simulink model "metab_platform"  (Simulink 7.5)
settings: Solver=ode45  StartTime=0.0  StopTime=struttura.simul  FixedStep=0.5  MaxStep=1  RelTol=1e-3
undefined symbols (not defined in the file or in its folder): hardware, struttura
settings Model: Creator=Marc Breton  LastModifiedBy=sriddle
settings SolverCC: InitialStep=0.5
settings DataIOCC: ExternalInput=[t,u]  LimitDataPoints=off  SaveOutput=off  SignalLogging=off  SaveTime=off
settings OptimizationCC: InitFltsAndDblsToZero=on
settings DebuggingCC: SaveWithParameterizedLinksMsg=none  SignalResolutionControl=TryResolveAllWithWarning  InheritedTsInSrcMsg=none  MultiTaskDSMMsg=warning  MultiTaskCondExecSysMsg=none  StrictBusMsg=Warning
settings RTWCC: IncludeERTFirstTime=on
settings GRTTargetCC: TargetFcnLib=ansi_tfl_tmw.mat

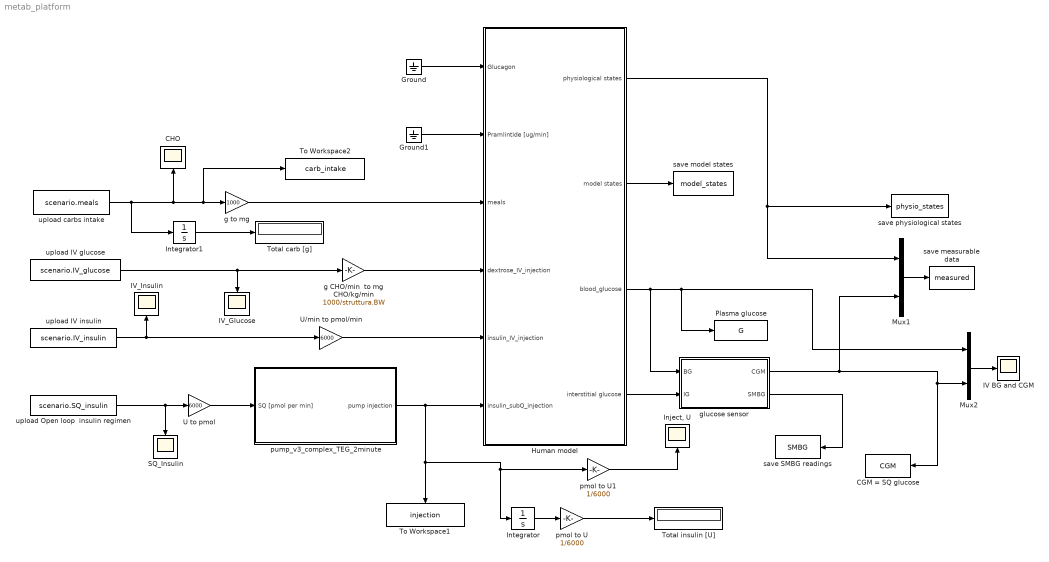
== system metab_platform ==
  CGM = SQ glucose : ToWorkspace  VariableName=CGM  SampleTime=-1  SaveFormat=Structure
  CHO : Scope
  Ground : Ground
  Ground1 : Ground
  Human model : Subsystem
  IV BG and CGM : Scope
      settings: YMin=0  YMax=3000
  IV_Glucose : Scope
      settings: YMin=-1  YMax=1  SaveName=ScopeData7
  IV_Insulin : Scope
      settings: YMin=-1  YMax=1  SaveName=ScopeData3
  "Inject, U" : Scope
      settings: SaveName=ScopeData2
  Integrator : Integrator
  Integrator1 : Integrator
  Mux1 : Mux  Inputs=2
  Mux2 : Mux  Inputs=2
  Plasma glucose : ToWorkspace  VariableName=G  SampleTime=-1  SaveFormat=Structure
  SQ_Insulin : Scope
      settings: SaveName=ScopeData6
  To Workspace1 : ToWorkspace  VariableName=injection  SampleTime=-1  SaveFormat=Structure
  To Workspace2 : ToWorkspace  VariableName=carb_intake  SampleTime=-1  SaveFormat=Structure
  Total carb [g] : Display
  Total insulin [U] : Display
  U to pmol : Gain  Gain=6000  ParameterDataType=sfix(16)  ParameterScaling=2^0  OutDataType=sfix(16)  OutScaling=2^0
  U/min to pmol/min : Gain  Gain=6000  ParameterDataType=sfix(16)  ParameterScaling=2^0  OutDataType=sfix(16)  OutScaling=2^0
  g CHO/min  to mg CHO/kg/min : Gain  Gain=1000/struttura.BW  ParameterDataType=sfix(16)  ParameterScaling=2^0  OutDataType=sfix(16)  OutScaling=2^0
  g to mg : Gain  Gain=1000  ParameterDataType=sfix(16)  ParameterScaling=2^0  OutDataType=sfix(16)  OutScaling=2^0
  glucose sensor : Subsystem
  pmol to U : Gain  Gain=1/6000  ParameterDataType=sfix(16)  ParameterScaling=2^0  OutDataType=sfix(16)  OutScaling=2^0
  pmol to U1 : Gain  Gain=1/6000  ParameterDataType=sfix(16)  ParameterScaling=2^0  OutDataType=sfix(16)  OutScaling=2^0
  pump_v3_complex_TEG_2minute : Subsystem
  save SMBG readings : ToWorkspace  VariableName=SMBG  SampleTime=-1  SaveFormat=Structure
  save measurable data : ToWorkspace  VariableName=measured  SampleTime=-1  SaveFormat=Structure
  save model states : ToWorkspace  VariableName=model_states  SampleTime=-1  SaveFormat=Structure With Time
  save physiological states : ToWorkspace  VariableName=physio_states  SampleTime=-1  SaveFormat=Structure With Time
  upload IV glucose : FromWorkspace  VariableName=scenario.IV_glucose  SampleTime=0
  upload IV insulin : FromWorkspace  VariableName=scenario.IV_insulin  SampleTime=0
  upload Open loop  insulin regimen : FromWorkspace  VariableName=scenario.SQ_insulin  SampleTime=0
  upload carbs intake : FromWorkspace  VariableName=scenario.meals  SampleTime=0
  wires:
  upload carbs intake/1 -> Integrator1/1, CHO/1, g to mg/1, To Workspace2/1
  g to mg/1 -> Human model/3(meals)
  upload Open loop  insulin regimen/1 -> U to pmol/1, SQ_Insulin/1
  U to pmol/1 -> pump_v3_complex_TEG_2minute/1(SQ [pmol per min])
  pump_v3_complex_TEG_2minute/1(pump injection) -> To Workspace1/1, Integrator/1, pmol to U1/1, Human model/6(insulin_subQ_injection)
  Integrator/1 -> pmol to U/1
  pmol to U/1 -> Total insulin [U]/1
  Integrator1/1 -> Total carb [g]/1
  upload IV glucose/1 -> g CHO/min  to mg CHO/kg/min/1, IV_Glucose/1
  upload IV insulin/1 -> U/min to pmol/min/1, IV_Insulin/1
  U/min to pmol/min/1 -> Human model/5(insulin_IV_injection)
  g CHO/min  to mg CHO/kg/min/1 -> Human model/4(dextrose_IV_injection)
  Human model/3(blood_glucose) -> Mux2/1, Plasma glucose/1, glucose sensor/1(BG)
  Human model/1(physiological states) -> Mux1/1, save physiological states/1
  Human model/2(model states) -> save model states/1
  Human model/4(interstitial glucose) -> glucose sensor/2(IG)
  Mux1/1 -> save measurable data/1
  glucose sensor/2(SMBG) -> save SMBG readings/1
  glucose sensor/1(CGM) -> Mux1/2, CGM = SQ glucose/1, Mux2/2
  Mux2/1 -> IV BG and CGM/1
  pmol to U1/1 -> "Inject, U"/1
  Ground/1 -> Human model/1(Glucagon)
  Ground1/1 -> Human model/2(Pramlintide [ug/min])

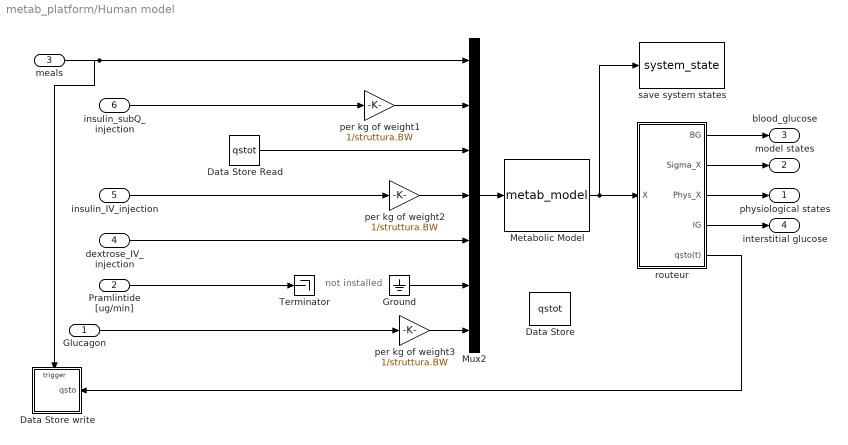
== system metab_platform/Human model ==
  note: not
      | installed
  Glucagon : Inport
  Pramlintide [ug/min] : Inport  Port=2
  meals : Inport  Port=3
  dextrose_IV_injection : Inport  Port=4
  insulin_IV_injection : Inport  Port=5
  insulin_subQ_injection : Inport  Port=6
  Data Store : DataStoreMemory  DataStoreName=qstot
  Data Store Read : DataStoreRead  DataStoreName=qstot  SampleTime=-1
  Data Store write : Subsystem  TreatAsAtomicUnit=on
  Ground : Ground
  Metabolic Model : S-Function  FunctionName=metab_model  Parameters=struttura  EnableBusSupport=off
  Mux2 : Mux  Inputs=7
  Terminator : Terminator
  per kg of weight1 : Gain  Gain=1/struttura.BW
  per kg of weight2 : Gain  Gain=1/struttura.BW
  per kg of weight3 : Gain  Gain=1/struttura.BW
  routeur : Subsystem
  save system states : ToWorkspace  VariableName=system_state  SampleTime=-1  SaveFormat=Structure With Time
  physiological states : Outport
  model states : Outport  Port=2
  blood_glucose : Outport  Port=3
  interstitial glucose : Outport  Port=4
  wires:
  Metabolic Model/1 -> routeur/1(X), save system states/1
  routeur/3(Phys_X) -> physiological states/1
  routeur/1(BG) -> blood_glucose/1
  insulin_subQ_injection/1 -> per kg of weight1/1
  Mux2/1 -> Metabolic Model/1
  routeur/2(Sigma_X) -> model states/1
  Data Store Read/1 -> Mux2/3
  routeur/4(IG) -> interstitial glucose/1
  per kg of weight1/1 -> Mux2/2
  insulin_IV_injection/1 -> per kg of weight2/1
  dextrose_IV_injection/1 -> Mux2/5
  routeur/5(qsto(t)) -> Data Store write/1(qsto)
  per kg of weight2/1 -> Mux2/4
  meals/1 -> Data Store write/Trigger, Mux2/1
  Pramlintide [ug/min]/1 -> Terminator/1
  Ground/1 -> Mux2/6
  Glucagon/1 -> per kg of weight3/1
  per kg of weight3/1 -> Mux2/7

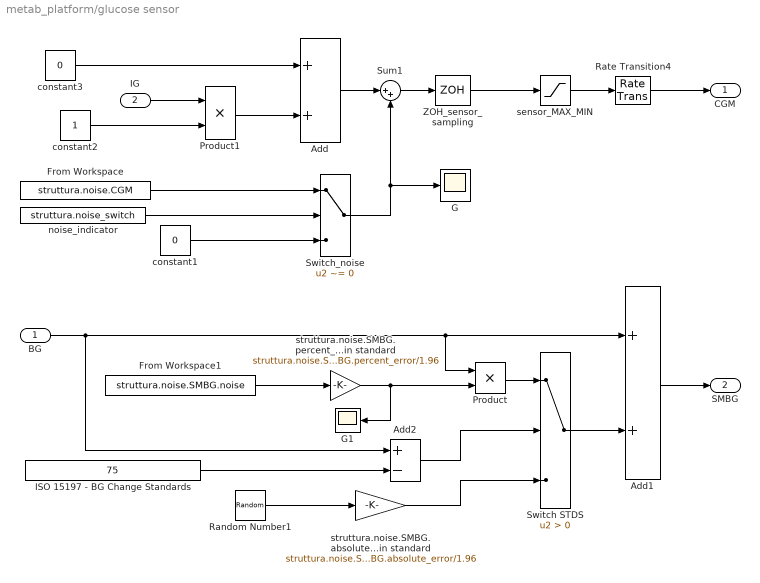
== system metab_platform/glucose sensor ==
  BG : Inport
  IG : Inport  Port=2
  Add : Sum
  Add1 : Sum
  Add2 : Sum  Inputs=+-
  From Workspace : FromWorkspace  VariableName=struttura.noise.CGM  SampleTime=0
  From Workspace1 : FromWorkspace  VariableName=struttura.noise.SMBG.noise  SampleTime=0
  G : Scope
      settings: YMin=-32.5  YMax=10  SaveName=ScopeData4
  G1 : Scope
      settings: YMin=-0.35  YMax=0.3  SaveName=ScopeData8
  ISO 15197 - BG Change Standards : Constant  Value=75
  Product : Product  RndMeth=Zero
  Product1 : Product  RndMeth=Zero
  Random Number1 : RandomNumber  Variance=0.2  Seed=1  SampleTime=1
  Rate Transition4 : RateTransition  X0=struttura.x0(4)/struttura.Vg  OutPortSampleTime=1
  Sum1 : Sum  Inputs=|++
  Switch STDS : Switch  Criteria=u2 > Threshold
  Switch_noise : Switch  Criteria=u2 ~= 0  Threshold=1440
  ZOH_sensor_sampling : ZeroOrderHold  SampleTime=hardware.sensor_sampling
  constant1 : Constant  Value=0
  constant2 : Constant
  constant3 : Constant  Value=0
  noise_indicator : Constant  Value=struttura.noise_switch
  sensor_MAX_MIN : Saturate  UpperLimit=hardware.sensor_max  LowerLimit=hardware.sensor_min
  struttura.noise.SMBG.absolute_error/1.96 95% of values to fall within standard : Gain  Gain=struttura.noise.SMBG.absolute_error/1.96
  struttura.noise.SMBG.percent_error/1.96 95% of values to fall within standard : Gain  Gain=struttura.noise.SMBG.percent_error/1.96
  CGM : Outport
  SMBG : Outport  Port=2
  wires:
  Sum1/1 -> ZOH_sensor_sampling/1
  ZOH_sensor_sampling/1 -> sensor_MAX_MIN/1
  sensor_MAX_MIN/1 -> Rate Transition4/1
  From Workspace/1 -> Switch_noise/1
  noise_indicator/1 -> Switch_noise/2
  constant1/1 -> Switch_noise/3
  Switch_noise/1 -> Sum1/2, G/1
  IG/1 -> Product1/1
  constant3/1 -> Add/1
  Product1/1 -> Add/2
  Add/1 -> Sum1/1
  Rate Transition4/1 -> CGM/1
  From Workspace1/1 -> struttura.noise.SMBG.percent_error/1.96 95% of values to fall within standard/1
  BG/1 -> Add2/1, Add1/1, Product/1
  ISO 15197 - BG Change Standards/1 -> Add2/2
  struttura.noise.SMBG.percent_error/1.96 95% of values to fall within standard/1 -> Product/2, G1/1
  Product/1 -> Switch STDS/1
  Switch STDS/1 -> Add1/2
  Add2/1 -> Switch STDS/2
  Random Number1/1 -> struttura.noise.SMBG.absolute_error/1.96 95% of values to fall within standard/1
  struttura.noise.SMBG.absolute_error/1.96 95% of values to fall within standard/1 -> Switch STDS/3
  Add1/1 -> SMBG/1
  constant2/1 -> Product1/2

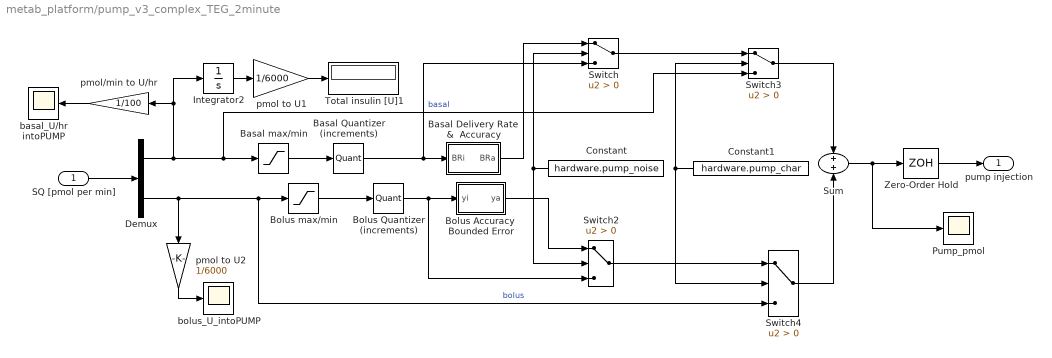
== system metab_platform/pump_v3_complex_TEG_2minute ==
  SQ [pmol per min] : Inport
  Basal Delivery Rate  &  Accuracy : Subsystem
  Basal Quantizer (increments) : Quantizer  QuantizationInterval=hardware.pump_basal_inc
  Basal max/min : Saturate  UpperLimit=hardware.pump_basal_max  LowerLimit=hardware.pump_basal_min
  Bolus Accuracy  Bounded Error : Subsystem
  Bolus Quantizer (increments) : Quantizer  QuantizationInterval=hardware.pump_bolus_inc
  Bolus max/min : Saturate  UpperLimit=hardware.pump_bolus_max  LowerLimit=0
  Constant : Constant  Value=hardware.pump_noise
  Constant1 : Constant  Value=hardware.pump_char
  Demux : Demux  Outputs=2
  Integrator2 : Integrator
  Pump_pmol : Scope
      settings: YMin=0  YMax=175  SaveName=ScopeData16
  Sum : Sum  Inputs=+|+
  Switch{,2..4} (4 alike) : Switch  Criteria=u2 > Threshold
  Total insulin [U]1 : Display
  Zero-Order Hold : ZeroOrderHold
  basal_U/hr intoPUMP : Scope
      settings: YMin=0  YMax=175  SaveName=ScopeData15
  bolus_U_intoPUMP : Scope
      settings: YMin=0  YMax=175  SaveName=ScopeData5
  pmol to U1 : Gain  Gain=1/6000
  pmol to U2 : Gain  Gain=1/6000
  pmol/min to U/hr : Gain  Gain=1/100
  pump injection : Outport
  wires:
  Zero-Order Hold/1 -> pump injection/1
  pmol to U1/1 -> Total insulin [U]1/1
  Integrator2/1 -> pmol to U1/1
  Bolus max/min/1 -> Bolus Quantizer (increments)/1
  SQ [pmol per min]/1 -> Demux/1
  Sum/1 -> Zero-Order Hold/1, Pump_pmol/1
  Demux/1 -> Basal max/min/1, Switch3/3, Integrator2/1, pmol/min to U/hr/1  "basal"
  Basal max/min/1 -> Basal Quantizer (increments)/1
  Demux/2 -> Bolus max/min/1, Switch4/3, pmol to U2/1  "bolus"
  Bolus Quantizer (increments)/1 -> Bolus Accuracy  Bounded Error/1(yi), Switch2/3
  Basal Quantizer (increments)/1 -> Basal Delivery Rate  &  Accuracy/1(BRi), Switch/3
  Basal Delivery Rate  &  Accuracy/1(BRa) -> Switch/1
  Constant/1 -> Switch2/2, Switch/2
  Bolus Accuracy  Bounded Error/1(ya) -> Switch2/1
  Switch2/1 -> Switch4/1
  Switch/1 -> Switch3/1
  Constant1/1 -> Switch4/2, Switch3/2
  Switch3/1 -> Sum/1
  Switch4/1 -> Sum/2
  pmol to U2/1 -> bolus_U_intoPUMP/1
  pmol/min to U/hr/1 -> basal_U/hr intoPUMP/1

== system metab_platform/Human model/Data Store write ==
  qsto : Inport  LatchByDelayingOutsideSignal=on
  Trigger : TriggerPort
  Data Store Write : DataStoreWrite  DataStoreName=qstot  SampleTime=-1
  wires:
  qsto/1 -> Data Store Write/1

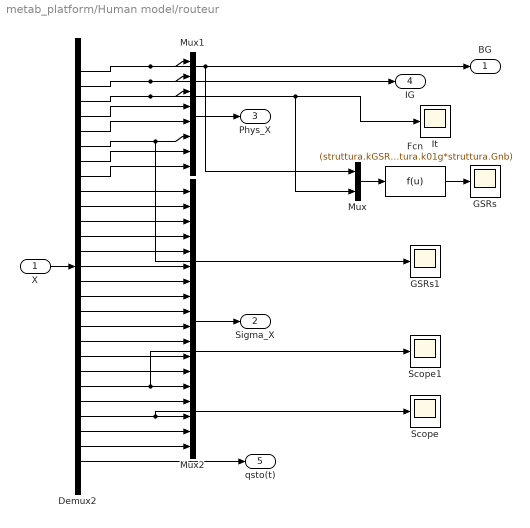
== system metab_platform/Human model/routeur ==
  X : Inport
  Demux2 : Demux  Outputs=27
  Fcn : Fcn  Expr=(struttura.kGSRs*(struttura.Gth-(u(1)))/((u(2)-struttura.Ith)+1)+struttura.k01g*struttura.Gnb)
  GSRs : Scope
      settings: SaveName=ScopeData13
  GSRs1 : Scope
      settings: SaveName=ScopeData14
  It : Scope
      settings: SaveName=ScopeData10
  Mux : Mux  Inputs=2
  Mux1 : Mux  Inputs=8
  Mux2 : Mux  Inputs=18
  Scope : Scope
  Scope1 : Scope
      settings: SaveName=ScopeData2
  BG : Outport
  Sigma_X : Outport  Port=2
  Phys_X : Outport  Port=3
  IG : Outport  Port=4
  qsto(t) : Outport  Port=5
  wires:
  X/1 -> Demux2/1
  Mux1/1 -> Phys_X/1
  Demux2/1 -> Mux1/1, BG/1, Mux/1
  Demux2/2 -> Mux1/2, IG/1
  Demux2/3 -> Mux1/3, It/1, Mux/2
  Demux2/4 -> Mux1/4
  Demux2/5 -> Mux1/5
  Demux2/6 -> Mux1/6, GSRs1/1
  Demux2/7 -> Mux1/7
  Demux2/8 -> Mux1/8
  Demux2/9 -> Mux2/1
  Demux2/10 -> Mux2/2
  Demux2/11 -> Mux2/3
  Demux2/12 -> Mux2/4
  Demux2/13 -> Mux2/5
  Demux2/14 -> Mux2/6
  Demux2/15 -> Mux2/7
  Demux2/16 -> Mux2/8
  Demux2/17 -> Mux2/9
  Demux2/18 -> Mux2/10
  Demux2/19 -> Mux2/11
  Mux2/1 -> Sigma_X/1
  Mux/1 -> Fcn/1
  Fcn/1 -> GSRs/1
  Demux2/27 -> qsto(t)/1
  Demux2/20 -> Mux2/12
  Demux2/21 -> Mux2/13
  Demux2/22 -> Scope1/1, Mux2/14
  Demux2/23 -> Mux2/15
  Demux2/24 -> Mux2/16, Scope/1
  Demux2/25 -> Mux2/17
  Demux2/26 -> Mux2/18

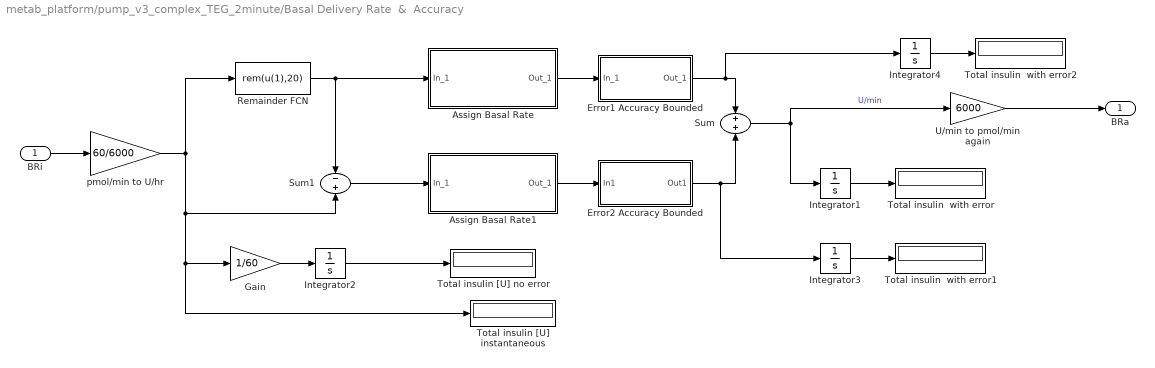
== system metab_platform/pump_v3_complex_TEG_2minute/Basal Delivery Rate  &  Accuracy ==
  BRi : Inport
  Assign Basal Rate : Subsystem
  Assign Basal Rate1 : Subsystem
  Error1 Accuracy Bounded : Subsystem
  Error2 Accuracy Bounded : Subsystem
  Gain : Gain  Gain=1/60
  Integrator{1..4} (4 alike) : Integrator
  Remainder FCN : Fcn  Expr=rem(u(1),20)
  Sum : Sum  Inputs=+|+
  Sum1 : Sum  Inputs=-|+
  Total insulin  with error : Display
  Total insulin  with error1 : Display
  Total insulin  with error2 : Display
  Total insulin [U] instantaneous : Display
  Total insulin [U] no error : Display
  U/min to pmol/min again : Gain  Gain=6000
  pmol/min to U/hr : Gain  Gain=60/6000
  BRa : Outport
  wires:
  Sum1/1 -> Assign Basal Rate1/1(In_1)
  Remainder FCN/1 -> Sum1/1, Assign Basal Rate/1(In_1)
  Integrator4/1 -> Total insulin  with error2/1
  Integrator3/1 -> Total insulin  with error1/1
  Sum/1 -> Integrator1/1, U/min to pmol/min again/1  "U/min"
  Error1 Accuracy Bounded/1(Out_1) -> Integrator4/1, Sum/1
  Assign Basal Rate/1(Out_1) -> Error1 Accuracy Bounded/1(In_1)
  Error2 Accuracy Bounded/1(Out1) -> Integrator3/1, Sum/2
  Assign Basal Rate1/1(Out_1) -> Error2 Accuracy Bounded/1(In1)
  Integrator2/1 -> Total insulin [U] no error/1
  Gain/1 -> Integrator2/1
  Integrator1/1 -> Total insulin  with error/1
  U/min to pmol/min again/1 -> BRa/1
  pmol/min to U/hr/1 -> Sum1/2, Total insulin [U] instantaneous/1, Gain/1, Remainder FCN/1
  BRi/1 -> pmol/min to U/hr/1

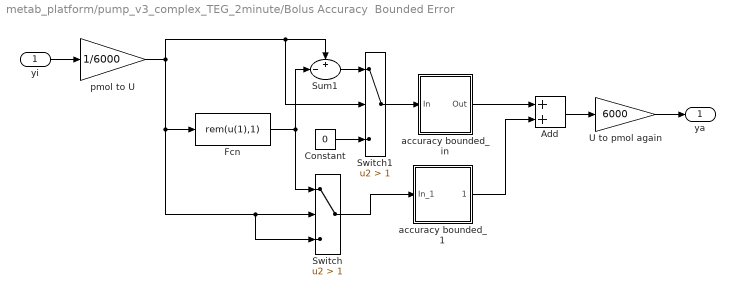
== system metab_platform/pump_v3_complex_TEG_2minute/Bolus Accuracy  Bounded Error ==
  yi : Inport
  Add : Sum
  Constant : Constant  Value=0
  Fcn : Fcn  Expr=rem(u(1),1)
  Sum1 : Sum  Inputs=+-|
  Switch : Switch  Criteria=u2 > Threshold  Threshold=1
  Switch1 : Switch  Criteria=u2 > Threshold  Threshold=1
  U to pmol again : Gain  Gain=6000
  accuracy bounded_1 : Subsystem
  accuracy bounded_in : Subsystem
  pmol to U : Gain  Gain=1/6000
  ya : Outport
  wires:
  Switch1/1 -> accuracy bounded_in/1(In)
  Constant/1 -> Switch1/3
  Sum1/1 -> Switch1/1
  Switch/1 -> accuracy bounded_1/1(In_1)
  Fcn/1 -> Sum1/2, Switch/1
  accuracy bounded_1/1(Out_1) -> Add/2
  accuracy bounded_in/1(Out) -> Add/1
  Add/1 -> U to pmol again/1
  U to pmol again/1 -> ya/1
  pmol to U/1 -> Switch1/2, Sum1/1, Switch/3, Switch/2, Fcn/1
  yi/1 -> pmol to U/1

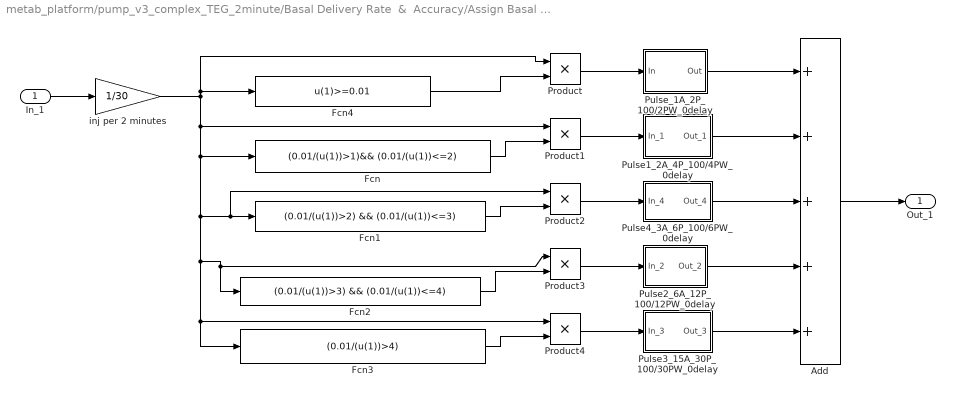
== system metab_platform/pump_v3_complex_TEG_2minute/Basal Delivery Rate  &  Accuracy/Assign Basal Rate ==
  In_1 : Inport
  Add : Sum  Inputs=+++++
  Fcn : Fcn  Expr=(0.01/(u(1))>1)&& (0.01/(u(1))<=2)
  Fcn1 : Fcn  Expr=(0.01/(u(1))>2) && (0.01/(u(1))<=3)
  Fcn2 : Fcn  Expr=(0.01/(u(1))>3) && (0.01/(u(1))<=4)
  Fcn3 : Fcn  Expr=(0.01/(u(1))>4)
  Fcn4 : Fcn  Expr=u(1)>=0.01
  Product{,1..4} (5 alike) : Product  RndMeth=Zero
  Pulse1_2A_4P_100/4PW_0delay : Subsystem
  Pulse2_6A_12P_100/12PW_0delay : Subsystem
  Pulse3_15A_30P_100/30PW_0delay : Subsystem
  Pulse4_3A_6P_100/6PW_0delay : Subsystem
  Pulse_1A_2P_100/2PW_0delay : Subsystem
  inj per 2 minutes : Gain  Gain=1/30
  Out_1 : Outport
  wires:
  inj per 2 minutes/1 -> Product/1, Fcn4/1, Fcn2/1, Product3/1, Fcn3/1, Product4/1, Fcn1/1, Product2/1, Fcn/1, Product1/1
  Add/1 -> Out_1/1
  Pulse3_15A_30P_100/30PW_0delay/1(Out_3) -> Add/5
  Pulse2_6A_12P_100/12PW_0delay/1(Out_2) -> Add/4
  Pulse4_3A_6P_100/6PW_0delay/1(Out_4) -> Add/3
  Pulse1_2A_4P_100/4PW_0delay/1(Out_1) -> Add/2
  Pulse_1A_2P_100/2PW_0delay/1(Out) -> Add/1
  Product1/1 -> Pulse1_2A_4P_100/4PW_0delay/1(In_1)
  Product2/1 -> Pulse4_3A_6P_100/6PW_0delay/1(In_4)
  Product3/1 -> Pulse2_6A_12P_100/12PW_0delay/1(In_2)
  Product4/1 -> Pulse3_15A_30P_100/30PW_0delay/1(In_3)
  Fcn3/1 -> Product4/2
  Fcn2/1 -> Product3/2
  Fcn1/1 -> Product2/2
  Fcn/1 -> Product1/2
  Fcn4/1 -> Product/2
  Product/1 -> Pulse_1A_2P_100/2PW_0delay/1(In)
  In_1/1 -> inj per 2 minutes/1

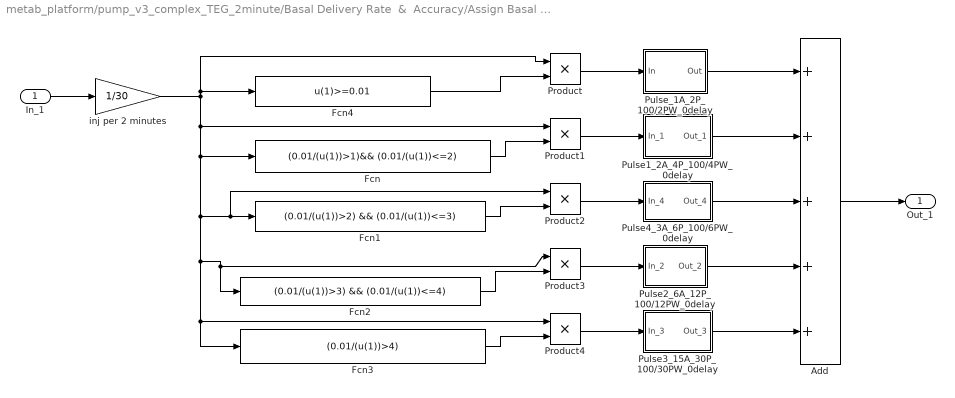
== system metab_platform/pump_v3_complex_TEG_2minute/Basal Delivery Rate  &  Accuracy/Assign Basal Rate1 ==
  In_1 : Inport
  Add : Sum  Inputs=+++++
  Fcn : Fcn  Expr=(0.01/(u(1))>1)&& (0.01/(u(1))<=2)
  Fcn1 : Fcn  Expr=(0.01/(u(1))>2) && (0.01/(u(1))<=3)
  Fcn2 : Fcn  Expr=(0.01/(u(1))>3) && (0.01/(u(1))<=4)
  Fcn3 : Fcn  Expr=(0.01/(u(1))>4)
  Fcn4 : Fcn  Expr=u(1)>=0.01
  Product{,1..4} (5 alike) : Product  RndMeth=Zero
  Pulse1_2A_4P_100/4PW_0delay : Subsystem
  Pulse2_6A_12P_100/12PW_0delay : Subsystem
  Pulse3_15A_30P_100/30PW_0delay : Subsystem
  Pulse4_3A_6P_100/6PW_0delay : Subsystem
  Pulse_1A_2P_100/2PW_0delay : Subsystem
  inj per 2 minutes : Gain  Gain=1/30
  Out_1 : Outport
  wires:
  inj per 2 minutes/1 -> Product/1, Fcn4/1, Fcn2/1, Product3/1, Fcn3/1, Product4/1, Fcn1/1, Product2/1, Fcn/1, Product1/1
  Add/1 -> Out_1/1
  Pulse3_15A_30P_100/30PW_0delay/1(Out_3) -> Add/5
  Pulse2_6A_12P_100/12PW_0delay/1(Out_2) -> Add/4
  Pulse4_3A_6P_100/6PW_0delay/1(Out_4) -> Add/3
  Pulse1_2A_4P_100/4PW_0delay/1(Out_1) -> Add/2
  Pulse_1A_2P_100/2PW_0delay/1(Out) -> Add/1
  Product1/1 -> Pulse1_2A_4P_100/4PW_0delay/1(In_1)
  Product2/1 -> Pulse4_3A_6P_100/6PW_0delay/1(In_4)
  Product3/1 -> Pulse2_6A_12P_100/12PW_0delay/1(In_2)
  Product4/1 -> Pulse3_15A_30P_100/30PW_0delay/1(In_3)
  Fcn3/1 -> Product4/2
  Fcn2/1 -> Product3/2
  Fcn1/1 -> Product2/2
  Fcn/1 -> Product1/2
  Fcn4/1 -> Product/2
  Product/1 -> Pulse_1A_2P_100/2PW_0delay/1(In)
  In_1/1 -> inj per 2 minutes/1

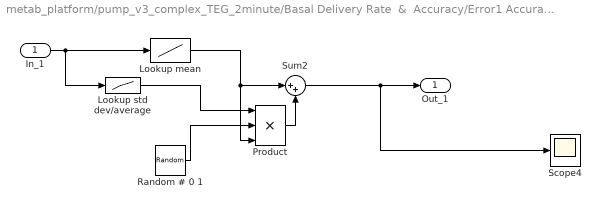
== system metab_platform/pump_v3_complex_TEG_2minute/Basal Delivery Rate  &  Accuracy/Error1 Accuracy Bounded ==
  In_1 : Inport
  Lookup mean : Lookup  InputValues=hardware.pump_accuracy_bolus_amount  Table=hardware.pump_bolus_mean
  Lookup std dev/average : Lookup  InputValues=hardware.pump_accuracy_bolus_amount  Table=hardware.pump_bolus_std2r
  Product : Product  Inputs=3  RndMeth=Zero
  "Random # 0 1 " : RandomNumber  SampleTime=1
  Scope4 : Scope
      settings: YMin=0  YMax=175  SaveName=ScopeData30
  Sum2 : Sum  Inputs=|++
  Out_1 : Outport
  wires:
  In_1/1 -> Lookup std dev/average/1, Lookup mean/1
  "Random # 0 1 "/1 -> Product/2
  Lookup std dev/average/1 -> Product/1
  Product/1 -> Sum2/2
  Sum2/1 -> Out_1/1, Scope4/1
  Lookup mean/1 -> Sum2/1, Product/3

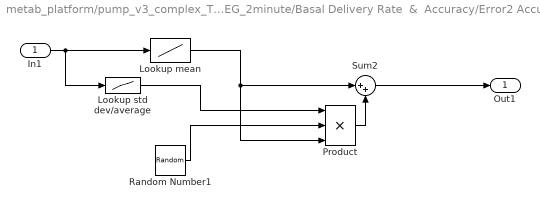
== system metab_platform/pump_v3_complex_TEG_2minute/Basal Delivery Rate  &  Accuracy/Error2 Accuracy Bounded ==
  In1 : Inport
  Lookup mean : Lookup  InputValues=hardware.pump_accuracy_bolus_amount  Table=hardware.pump_bolus_mean
  Lookup std dev/average : Lookup  InputValues=hardware.pump_accuracy_bolus_amount  Table=hardware.pump_bolus_std2r
  Product : Product  Inputs=3  RndMeth=Zero
  Random Number1 : RandomNumber  SampleTime=1
  Sum2 : Sum  Inputs=|++
  Out1 : Outport
  wires:
  Lookup mean/1 -> Product/3, Sum2/1
  Sum2/1 -> Out1/1
  Product/1 -> Sum2/2
  Lookup std dev/average/1 -> Product/1
  Random Number1/1 -> Product/2
  In1/1 -> Lookup mean/1, Lookup std dev/average/1

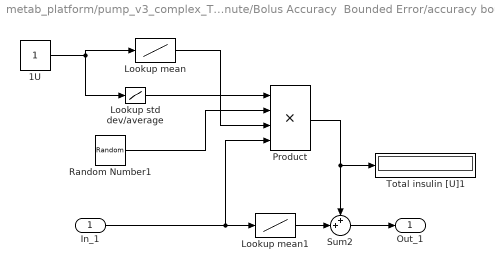
== system metab_platform/pump_v3_complex_TEG_2minute/Bolus Accuracy  Bounded Error/accuracy bounded_1 ==
  In_1 : Inport
  1U : Constant
  Lookup mean : Lookup  InputValues=hardware.pump_accuracy_bolus_amount  Table=hardware.pump_bolus_mean  LookUpMeth=Interpolation-Use End Values
  Lookup mean1 : Lookup  InputValues=hardware.pump_accuracy_bolus_amount  Table=hardware.pump_bolus_mean
  Lookup std dev/average : Lookup  InputValues=hardware.pump_accuracy_bolus_amount  Table=hardware.pump_bolus_std2r  LookUpMeth=Interpolation-Use End Values
  Product : Product  Inputs=4  RndMeth=Zero
  Random Number1 : RandomNumber  SampleTime=1
  Sum2 : Sum  Inputs=++|
  Total insulin [U]1 : Display
  Out_1 : Outport
  wires:
  Lookup std dev/average/1 -> Product/1
  Product/1 -> Total insulin [U]1/1, Sum2/1
  Lookup mean1/1 -> Sum2/2
  In_1/1 -> Lookup mean1/1, Product/4
  1U/1 -> Lookup std dev/average/1, Lookup mean/1
  Random Number1/1 -> Product/2
  Lookup mean/1 -> Product/3
  Sum2/1 -> Out_1/1

== system metab_platform/pump_v3_complex_TEG_2minute/Bolus Accuracy  Bounded Error/accuracy bounded_in ==
  In : Inport
  Lookup mean : Lookup  InputValues=hardware.pump_accuracy_bolus_amount  Table=hardware.pump_bolus_mean
  Lookup std dev/average : Lookup  InputValues=hardware.pump_accuracy_bolus_amount  Table=hardware.pump_bolus_std2r  LookUpMeth=Interpolation-Use End Values
  Product : Product  Inputs=3  RndMeth=Zero
  Random Number1 : RandomNumber  SampleTime=1
  Sum2 : Sum  Inputs=|++
  Out : Outport
  wires:
  Sum2/1 -> Out/1
  In/1 -> Lookup mean/1, Lookup std dev/average/1
  Product/1 -> Sum2/2
  Lookup mean/1 -> Product/3, Sum2/1
  Lookup std dev/average/1 -> Product/1
  Random Number1/1 -> Product/2

== system metab_platform/pump_v3_complex_TEG_2minute/Basal Delivery Rate  &  Accuracy/Assign Basal Rate/Pulse1_2A_4P_100/4PW_0delay ==
  In_1 : Inport
  Product1 : Product  RndMeth=Zero
  Pulse Generator : DiscretePulseGenerator  PulseType=Time based  Amplitude=2  Period=4  PulseWidth=100/4  PhaseDelay=0  SampleTime=1
  Out_1 : Outport
  wires:
  Pulse Generator/1 -> Product1/2
  Product1/1 -> Out_1/1
  In_1/1 -> Product1/1

== system metab_platform/pump_v3_complex_TEG_2minute/Basal Delivery Rate  &  Accuracy/Assign Basal Rate/Pulse2_6A_12P_100/12PW_0delay ==
  In_2 : Inport
  Product1 : Product  RndMeth=Zero
  Pulse Generator : DiscretePulseGenerator  PulseType=Time based  Amplitude=6  Period=12  PulseWidth=100/12  PhaseDelay=0  SampleTime=1
  Out_2 : Outport
  wires:
  Product1/1 -> Out_2/1
  In_2/1 -> Product1/1
  Pulse Generator/1 -> Product1/2

== system metab_platform/pump_v3_complex_TEG_2minute/Basal Delivery Rate  &  Accuracy/Assign Basal Rate/Pulse3_15A_30P_100/30PW_0delay ==
  In_3 : Inport
  Product1 : Product  RndMeth=Zero
  Pulse Generator : DiscretePulseGenerator  PulseType=Time based  Amplitude=15  Period=30  PulseWidth=100/30  PhaseDelay=0  SampleTime=1
  Out_3 : Outport
  wires:
  Product1/1 -> Out_3/1
  In_3/1 -> Product1/1
  Pulse Generator/1 -> Product1/2

== system metab_platform/pump_v3_complex_TEG_2minute/Basal Delivery Rate  &  Accuracy/Assign Basal Rate/Pulse4_3A_6P_100/6PW_0delay ==
  In_4 : Inport
  Product1 : Product  RndMeth=Zero
  Pulse Generator : DiscretePulseGenerator  PulseType=Time based  Amplitude=3  Period=6  PulseWidth=100/6  PhaseDelay=0  SampleTime=1
  Out_4 : Outport
  wires:
  Product1/1 -> Out_4/1
  In_4/1 -> Product1/1
  Pulse Generator/1 -> Product1/2

== system metab_platform/pump_v3_complex_TEG_2minute/Basal Delivery Rate  &  Accuracy/Assign Basal Rate/Pulse_1A_2P_100/2PW_0delay ==
  In : Inport
  Product1 : Product  RndMeth=Zero
  Pulse Generator : DiscretePulseGenerator  PulseType=Time based  Amplitude=1  Period=2  PulseWidth=100/2  PhaseDelay=0  SampleTime=1
  Out : Outport
  wires:
  Product1/1 -> Out/1
  In/1 -> Product1/1
  Pulse Generator/1 -> Product1/2

== system metab_platform/pump_v3_complex_TEG_2minute/Basal Delivery Rate  &  Accuracy/Assign Basal Rate1/Pulse1_2A_4P_100/4PW_0delay ==
  In_1 : Inport
  Product1 : Product  RndMeth=Zero
  Pulse Generator : DiscretePulseGenerator  PulseType=Time based  Amplitude=2  Period=4  PulseWidth=100/4  PhaseDelay=0  SampleTime=1
  Out_1 : Outport
  wires:
  Pulse Generator/1 -> Product1/2
  Product1/1 -> Out_1/1
  In_1/1 -> Product1/1

== system metab_platform/pump_v3_complex_TEG_2minute/Basal Delivery Rate  &  Accuracy/Assign Basal Rate1/Pulse2_6A_12P_100/12PW_0delay ==
  In_2 : Inport
  Product1 : Product  RndMeth=Zero
  Pulse Generator : DiscretePulseGenerator  PulseType=Time based  Amplitude=6  Period=12  PulseWidth=100/12  PhaseDelay=0  SampleTime=1
  Out_2 : Outport
  wires:
  Product1/1 -> Out_2/1
  In_2/1 -> Product1/1
  Pulse Generator/1 -> Product1/2

== system metab_platform/pump_v3_complex_TEG_2minute/Basal Delivery Rate  &  Accuracy/Assign Basal Rate1/Pulse3_15A_30P_100/30PW_0delay ==
  In_3 : Inport
  Product1 : Product  RndMeth=Zero
  Pulse Generator : DiscretePulseGenerator  PulseType=Time based  Amplitude=15  Period=30  PulseWidth=100/30  PhaseDelay=0  SampleTime=1
  Out_3 : Outport
  wires:
  Product1/1 -> Out_3/1
  In_3/1 -> Product1/1
  Pulse Generator/1 -> Product1/2

== system metab_platform/pump_v3_complex_TEG_2minute/Basal Delivery Rate  &  Accuracy/Assign Basal Rate1/Pulse4_3A_6P_100/6PW_0delay ==
  In_4 : Inport
  Product1 : Product  RndMeth=Zero
  Pulse Generator : DiscretePulseGenerator  PulseType=Time based  Amplitude=3  Period=6  PulseWidth=100/6  PhaseDelay=0  SampleTime=1
  Out_4 : Outport
  wires:
  Product1/1 -> Out_4/1
  In_4/1 -> Product1/1
  Pulse Generator/1 -> Product1/2

== system metab_platform/pump_v3_complex_TEG_2minute/Basal Delivery Rate  &  Accuracy/Assign Basal Rate1/Pulse_1A_2P_100/2PW_0delay ==
  In : Inport
  Product1 : Product  RndMeth=Zero
  Pulse Generator : DiscretePulseGenerator  PulseType=Time based  Amplitude=1  Period=2  PulseWidth=100/2  PhaseDelay=0  SampleTime=1
  Out : Outport
  wires:
  Product1/1 -> Out/1
  In/1 -> Product1/1
  Pulse Generator/1 -> Product1/2
